simulink model "oto_ramp_simu"  (R2020a)
settings: Solver=VariableStepAuto  StartTime=0.0  StopTime=10.0  MaxStep=0.001  RelTol=1e-3
InitFcn:
  | g=9.81;
  | kp=0.35;
  | f=2;
  | l=0.75;
  | kc=0.35;
settings Model: Creator=UBY 00  LastModifiedBy=UBY 00

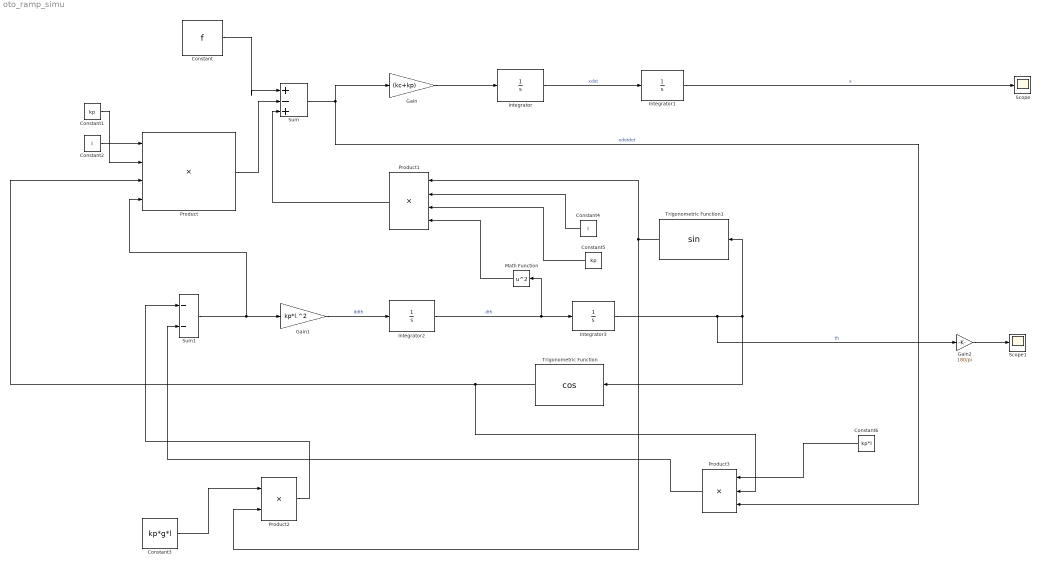
== system oto_ramp_simu ==
  Constant : Constant  Value=f
  Constant1 : Constant  Value=kp
  Constant2 : Constant  Value=l
  Constant3 : Constant  Value=kp*g*l
  Constant4 : Constant  Value=l
  Constant5 : Constant  Value=kp
  Constant6 : Constant  Value=kp*l
  Gain : Gain  Gain=(kc+kp)
  Gain1 : Gain  Gain=kp*l.^2
  Gain2 : Gain  Gain=180/pi
  Integrator : Integrator
  Integrator1 : Integrator  InitialCondition=0.15
  Integrator2 : Integrator
  Integrator3 : Integrator  InitialCondition=pi/3
  Math Function : Math  Operator=square  SaturateOnIntegerOverflow=on
  Product : Product  Inputs=4
  Product1 : Product  Inputs=4
  Product2 : Product
  Product3 : Product  Inputs=3
  Scope : Scope
  Scope1 : Scope
  Sum : Sum  Inputs=|+-+
  Sum1 : Sum  Inputs=--
  Trigonometric Function : Trigonometry  Operator=cos
  Trigonometric Function1 : Trigonometry
  wires:
  Integrator/1 -> Integrator1/1  "xdot"
  Integrator2/1 -> Math Function/1, Integrator3/1  "dth"
  Gain/1 -> Integrator/1
  Sum/1 -> Product3/3, Gain/1  "xdotdot"
  Integrator1/1 -> Scope/1  "x"
  Constant/1 -> Sum/1
  Gain1/1 -> Integrator2/1  "ddth"
  Integrator3/1 -> Gain2/1, Trigonometric Function/1, Trigonometric Function1/1  "th"
  Trigonometric Function/1 -> Product3/2, Product/3
  Constant2/1 -> Product/1
  Constant1/1 -> Product/2
  Sum1/1 -> Product/4, Gain1/1
  Trigonometric Function1/1 -> Product2/2, Product1/1
  Constant4/1 -> Product1/2
  Constant5/1 -> Product1/3
  Math Function/1 -> Product1/4
  Product/1 -> Sum/2
  Product1/1 -> Sum/3
  Constant3/1 -> Product2/1
  Product2/1 -> Sum1/1
  Constant6/1 -> Product3/1
  Product3/1 -> Sum1/2
  Gain2/1 -> Scope1/1
